simulink model "heli_day4_2"  (R2020b)
settings: Solver=ode1  StartTime=0.0  StopTime=20  FixedStep=0.002  RelTol=1e-3  EnableMultiTasking=on
PostLoadFcn:
  | qc_set_target_type(getConfigSet(bdroot, 'QUARC Default Target Configuration'));
undefined symbols (not defined in the file or in its folder): A_d, B_d, C_d, F, HIL, Joystick_gain_x, Joystick_gain_y, K, Q_d, qc_get_step_size, R_d
libraries: quarc_library x9
settings Model: SimulationMode=external  ExtModeTrigDuration=5000  Creator=Rchan  LastModifiedBy=endreeg
settings SolverCC: PositivePriorityOrder=on
settings DataIOCC: LimitDataPoints=on  SaveFormat=Array  SignalLoggingSaveFormat=ModelDataLogs  ReturnWorkspaceOutputs=off
settings OptimizationCC: ExpressionDepthLimit=2147483647  InitFltsAndDblsToZero=on  LifeSpan=inf
settings DebuggingCC: SaveWithParameterizedLinksMsg=none  UnderspecifiedInitializationDetection=Classic  MergeDetectMultiDrivingBlocksExec=none  SolverPrmCheckMsg=warning  MultiTaskDSMMsg=warning  MultiTaskCondExecSysMsg=none  FcnCallInpInsideContextMsg=warning  AllowSymbolicDim=off  StateNameClashWarn=warning  SFUnexpectedBacktrackingDiag=warning  SFNoUnconditionalDefaultTransitionDiag=warning  SFExecutionAtInitializationDiag=none  ArithmeticOperatorsInVariantConditions=warning
settings HardwareCC: ProdBitPerPointer=32  ProdBitPerSizeT=32  ProdBitPerPtrDiffT=32  ProdLargestAtomicFloat=None  ProdIntDivRoundTo=Undefined  ProdEndianess=Unspecified  ProdWordSize=32  ProdHWDeviceType=32-bit Generic
settings ModelReferenceCC: PropagateSignalLabelsOutOfModel=off
settings SFSimCC: SimUseLocalCustomCode=off  CustomCodeUndefinedFunction=UseInterfaceOnly
settings RTWCC: Description=QUARC Win64 Target  SystemTargetFile=quarc_win64.tlc  TemplateMakefile=quarc_default_tmf  RTWUseLocalCustomCode=off
settings CodeAppCC: StateflowObjectComments=on
settings GRTTargetCC: TargetLangStandard=C89/C90 (ANSI)  ParMdlRefBuildCompliant=off  CompOptLevelCompliant=off  CombineOutputUpdateFcns=off  MatFileLogging=off  GRTInterface=on  UseToolchainInfoCompliant=off  ExtMode=on  ExtModeMexFile=quarc_comm
settings ConfigComp: CovMetricSettings=dw  CovSaveCumulativeToWorkspaceVar=on  CovSaveSingleToWorkspaceVar=on  CovExternalEMLEnable=off  CovSFcnEnable=off

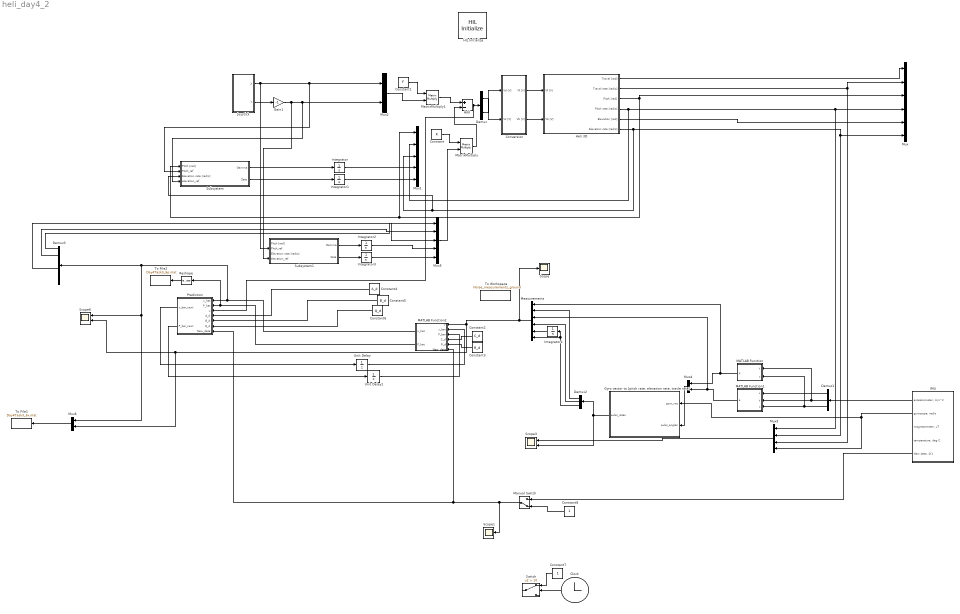
== system heli_day4_2 ==
  Add : Sum  Inputs=+-
  Clock : Clock
  Constant : Constant  Value=K
  Constant1 : Constant  Value=F
  Constant2 : Constant  Value=C_d
  Constant3 : Constant  Value=R_d
  Constant4 : Constant  Value=A_d
  Constant5 : Constant  Value=B_d
  Constant6 : Constant  Value=Q_d
  Constant7 : Constant
  Constant8 : Constant
  Conversion : Subsystem
  Demux : Demux  Outputs=2
  Demux1 : Demux  Outputs=3
  Demux2 : Demux  Outputs=3
  Demux3 : Demux  Outputs=6
  Gain1 : Gain  Gain=-1
  "Gyro vector to [pitch rate, elevation rate, travle rate]" : MATLAB Function  TreatAsAtomicUnit=on
  HIL Initialize : quarc_library/Data Acquisition/Generic/Configuration/HIL Initialize  Priority=-99  object_name=HIL-1  board_type=q8_usb  board_number=0  board_options=update_rate=normal;decimation=1  exclusive=off  active=off  hardware_clocks=[0:2]  clock_modes=[]  initial_clock_frequencies=[]  set_clock_params_at_start=off  set_clock_params_at_switch_in=off  set_clock_frequencies_at_start=off  set_clock_frequencies_at_switch_in=off  analog_input_channels=[0:7]  analog_input_configurations=[]  analog_input_maximums=10  analog_input_minimums=-10  set_analog_input_params_at_start=on  set_analog_input_params_at_switch_in=off  analog_output_channels=[0:7]  analog_output_maximums=10  analog_output_minimums=-10  initial_analog_outputs=[0]  final_analog_outputs=[0]  watchdog_analog_outputs=0  set_analog_output_params_at_start=on  set_analog_output_params_at_switch_in=off  set_analog_outputs_at_start=on  set_analog_outputs_at_switch_in=off  set_analog_outputs_at_terminate=on  set_analog_outputs_at_switch_out=off  set_analog_outputs_on_watchdog=off  digital_input_channels=[]  digital_output_channels=[]  digital_output_configuration=[]  initial_digital_outputs=[1]  final_digital_outputs=[1]  watchdog_digital_outputs=[1]  set_digital_output_params_at_start=off  set_digital_output_params_at_switch_in=off  set_digital_outputs_at_start=on  set_digital_outputs_at_switch_in=off  set_digital_outputs_at_terminate=on  set_digital_outputs_at_switch_out=off  set_digital_outputs_on_watchdog=off  encoder_channels=[0:7]  quadrature=[4]  encoder_filter_frequency=[]  initial_encoder_counts=[0]  set_encoder_params_at_start=on  set_encoder_params_at_switch_in=off  set_encoder_counts_at_start=on  set_encoder_counts_at_switch_in=off  pwm_channels=[0:7]  pwm_modes=0  pwm_frequency=99.532799999999995e6/4095  pwm_configuration=[0]  pwm_alignment=[0]  pwm_polarity=[1]  pwm_leading_deadband=[0]  pwm_trailing_deadband=[0]  initial_pwm_outputs=[0]  final_pwm_outputs=[0]  watchdog_pwm_outputs=[0]  set_pwm_params_at_start=on  set_pwm_params_at_switch_in=off  set_pwm_outputs_at_start=on  set_pwm_outputs_at_switch_in=off  set_pwm_outputs_at_terminate=on  set_pwm_outputs_at_switch_out=off  set_pwm_outputs_on_watchdog=off  other_output_channels=[]  initial_other_outputs=[]  final_other_outputs=[]  watchdog_other_outputs=[]  set_other_outputs_at_start=off  set_other_outputs_at_switch_in=off  set_other_outputs_at_terminate=off  set_other_outputs_at_switch_out=off  set_other_outputs_on_watchdog=off
  Heli 3D : Subsystem
  IMU : Subsystem
  Integrator{,1..4} (5 alike) : Integrator
  Joystick : Subsystem
  MATLAB Function : MATLAB Function  TreatAsAtomicUnit=on
  MATLAB Function1 : MATLAB Function  TreatAsAtomicUnit=on
  MATLAB Function2 : MATLAB Function  TreatAsAtomicUnit=on
  Manual Switch : ManualSwitch  CurrentSetting=0
  MatrixMultiply : Product  Multiplication=Matrix(*)
  MatrixMultiply1 : Product  Multiplication=Matrix(*)
  Measurements : Mux  Inputs=6
  Mux : Mux  Inputs=6
  Mux1 : Mux  Inputs=5
  Mux2 : Mux  Inputs=2
  Mux3 : Mux
  Mux4 : Mux  Inputs=2
  Mux5 : Mux  Inputs=5
  Mux6 : Mux  Inputs=2
  Prediction : MATLAB Function  TreatAsAtomicUnit=on
  Reshape : Reshape
  Scope : Scope
  Scope1 : Scope
  Scope3 : Scope  NumInputPorts=2
  Scope6 : Scope  NumInputPorts=2
  Subsystem : Subsystem
  Subsystem1 : Subsystem
  Switch : Switch  Criteria=u2 > Threshold  Threshold=10
  To File1 : ToFile  Filename=Day4Task3_6x.mat
  To File2 : ToFile  Filename=Day4Task3_6p.mat
  To Workspace : ToWorkspace  VariableName=Noise_measurements_ground  SampleTime=-1
  Unit Delay : UnitDelay  InitialCondition=[0,0,-0.5,0,0,0]  SampleTime=-1  HasFrameUpgradeWarning=on
  Unit Delay1 : UnitDelay  InitialCondition=eye(6)  SampleTime=-1  HasFrameUpgradeWarning=on
  wires:
  Heli 3D/1(Travel [rad]) -> Mux/1
  Heli 3D/2(Travel rate [rad/s]) -> Mux3/3, Mux/2
  Heli 3D/3(Pitch [rad]) -> Mux1/1, Subsystem/1(Pitch [rad]), Mux/3
  Heli 3D/4(Pitch rate [rad/s]) -> Mux3/1, Mux/4, Mux1/2
  Heli 3D/6(Elevation rate [rad/s]) -> Mux3/2, Mux/6, Mux1/3, Subsystem/3(Elevation rate [rad/s])
  Gain1/1 -> Mux2/2, Subsystem/4(elevation_ref), Subsystem1/4(elevation_ref)
  Joystick/2(Y) -> Gain1/1
  Demux/2 -> Conversion/1(Vd [V])
  MatrixMultiply/1 -> Add/2
  MatrixMultiply1/1 -> Add/1
  Constant/1 -> MatrixMultiply/1
  Constant1/1 -> MatrixMultiply1/1
  Mux2/1 -> MatrixMultiply1/2
  Demux/1 -> Conversion/2(Vs [V])
  Subsystem/1(Gamma) -> Integrator/1
  Integrator/1 -> Mux1/4
  Subsystem/2(Zeta) -> Integrator1/1
  Integrator1/1 -> Mux1/5
  Joystick/1(X) -> Mux2/1, Subsystem/2(Pitch_ref), Subsystem1/2(Pitch_ref)
  IMU/2("gyroscope, rad/s") -> "Gyro vector to [pitch rate, elevation rate, travle rate]"/1(gyro_vec), Mux3/4
  Mux3/1 -> Scope3/1
  IMU/1("accelerometer, m/s^2") -> Demux1/1
  Heli 3D/5(Elevation [rad]) -> Mux/5
  Mux4/1 -> "Gyro vector to [pitch rate, elevation rate, travle rate]"/2(euler_angles)
  MATLAB Function/1(p) -> Measurements/1, Mux4/1
  MATLAB Function1/1(e) -> Measurements/3, Mux4/2
  "Gyro vector to [pitch rate, elevation rate, travle rate]"/1(euler_rates) -> Demux2/1, Scope3/2
  Conversion/2(Vb [V]) -> Heli 3D/2(Vb [V])
  Conversion/1(Vf [V]) -> Heli 3D/1(Vf [V])
  Demux1/1 -> MATLAB Function1/1(x)
  Demux1/2 -> MATLAB Function/1(y), MATLAB Function1/2(y)
  Demux1/3 -> MATLAB Function/2(z), MATLAB Function1/3(z)
  Demux2/1 -> Measurements/2
  Demux2/2 -> Measurements/4
  Demux2/3 -> Measurements/6, Integrator4/1
  Subsystem1/1(Gamma) -> Integrator2/1
  Subsystem1/2(Zeta) -> Integrator3/1
  Integrator2/1 -> Mux5/4
  Integrator3/1 -> Mux5/5
  Demux3/1 -> Mux5/1
  Demux3/4 -> Mux5/3
  Demux3/2 -> Mux5/2
  Mux5/1 -> MatrixMultiply/2
  Mux6/1 -> To File1/1
  Integrator4/1 -> Measurements/5
  Measurements/1 -> Scope/1, MATLAB Function2/1(y), Mux6/2, Scope6/2
  Prediction/2(P_bar_next) -> Unit Delay1/1
  Constant2/1 -> MATLAB Function2/4(C_d)
  Constant3/1 -> MATLAB Function2/5(R_d)
  Unit Delay/1 -> MATLAB Function2/2(x_bar)
  Unit Delay1/1 -> MATLAB Function2/3(P_bar)
  Constant4/1 -> Prediction/4(A_d)
  Constant5/1 -> Prediction/5(B_d)
  Constant6/1 -> Prediction/6(Q_d)
  Prediction/1(x_bar_next) -> Unit Delay/1
  Add/1 -> Prediction/3(u), Demux/1
  MATLAB Function2/1(x_hat) -> Mux6/1, Scope6/1, Demux3/1, Prediction/1(x_hat)
  MATLAB Function2/2(P_hat) -> Reshape/1, Prediction/2(P_hat)
  Clock/1 -> Switch/2
  Constant7/1 -> Switch/1
  Constant8/1 -> Manual Switch/2
  IMU/5("New data, 0/1") -> Manual Switch/1
  Manual Switch/1 -> Scope1/1, Prediction/7(New_data), MATLAB Function2/6(New_data)
  Reshape/1 -> To File2/1

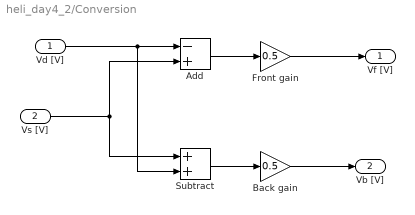
== system heli_day4_2/Conversion ==
  Vd [V] : Inport
  Vs [V] : Inport  Port=2
  Add : Sum  Inputs=-+
  Back gain : Gain  Gain=0.5
  Front gain : Gain  Gain=0.5
  Subtract : Sum
  Vf [V] : Outport
  Vb [V] : Outport  Port=2
  wires:
  Vd [V]/1 -> Subtract/2, Add/1
  Vs [V]/1 -> Add/2, Subtract/1
  Subtract/1 -> Back gain/1
  Back gain/1 -> Vb [V]/1
  Add/1 -> Front gain/1
  Front gain/1 -> Vf [V]/1

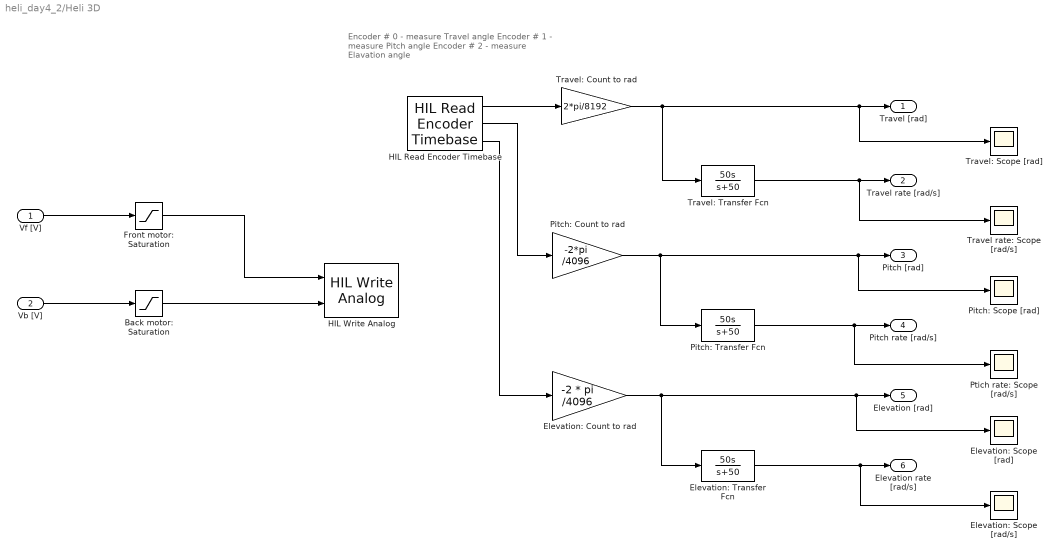
== system heli_day4_2/Heli 3D ==
  note: Encoder # 0 - measure Travel angle
      | Encoder # 1 - measure Pitch angle
      | Encoder # 2 - measure Elavation angle
  Vf [V] : Inport
  Vb [V] : Inport  Port=2
  Back motor: Saturation : Saturate  UpperLimit=5  LowerLimit=-5
  Elevation: Count to rad : Gain  Gain=-2 * pi /4096
  Elevation: Scope [rad/s] : Scope
  Elevation: Scope [rad] : Scope
  Elevation: Transfer Fcn : TransferFcn  Numerator=[50 0]  Denominator=[1 50]
  Front motor: Saturation : Saturate  UpperLimit=5  LowerLimit=-5
  HIL Read Encoder Timebase : quarc_library/Data Acquisition/Generic/Timebases/HIL Read Encoder Timebase  object_name=HIL-1  clock=0  channels=[0:2]  active=on  vector_output=off  data_type_mode=Inherit via back propagation  data_type=double  overflow_mode=Error on overflow  samples_in_buffer=max(ceil(1/qc_get_step_size), 1)
  HIL Write Analog : quarc_library/Data Acquisition/Generic/Immediate I//O/HIL Write Analog  object_name=HIL-1  channels=[0:1]  sample_time=-1  active=off  vector_input=off
  Pitch: Count to rad : Gain  Gain=-2*pi /4096
  Pitch: Scope [rad] : Scope
  Pitch: Transfer Fcn : TransferFcn  Numerator=[50 0]  Denominator=[1 50]
  Ptich rate: Scope [rad/s] : Scope
  Travel rate: Scope [rad/s] : Scope
  Travel: Count to rad : Gain  Gain=2*pi/8192
  Travel: Scope [rad] : Scope
  Travel: Transfer Fcn : TransferFcn  Numerator=[50 0]  Denominator=[1 50]
  Travel [rad] : Outport
  Travel rate [rad/s] : Outport  Port=2
  Pitch [rad] : Outport  Port=3
  Pitch rate [rad/s] : Outport  Port=4
  Elevation [rad] : Outport  Port=5
  Elevation rate [rad/s] : Outport  Port=6
  wires:
  HIL Read Encoder Timebase/1 -> Travel: Count to rad/1
  HIL Read Encoder Timebase/2 -> Pitch: Count to rad/1
  HIL Read Encoder Timebase/3 -> Elevation: Count to rad/1
  Travel: Count to rad/1 -> Travel: Scope [rad]/1, Travel [rad]/1, Travel: Transfer Fcn/1
  Travel: Transfer Fcn/1 -> Travel rate: Scope [rad/s]/1, Travel rate [rad/s]/1
  Pitch: Count to rad/1 -> Pitch: Transfer Fcn/1, Pitch: Scope [rad]/1, Pitch [rad]/1
  Pitch: Transfer Fcn/1 -> Ptich rate: Scope [rad/s]/1, Pitch rate [rad/s]/1
  Elevation: Count to rad/1 -> Elevation: Transfer Fcn/1, Elevation: Scope [rad]/1, Elevation [rad]/1
  Elevation: Transfer Fcn/1 -> Elevation: Scope [rad/s]/1, Elevation rate [rad/s]/1
  Vf [V]/1 -> Front motor: Saturation/1
  Vb [V]/1 -> Back motor: Saturation/1
  Front motor: Saturation/1 -> HIL Write Analog/1
  Back motor: Saturation/1 -> HIL Write Analog/2

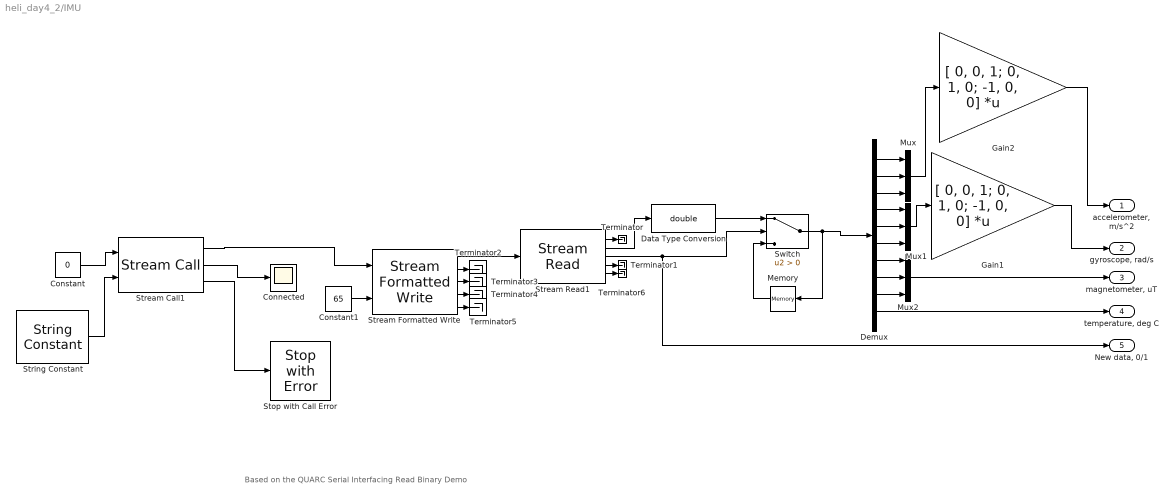
== system heli_day4_2/IMU ==
  note: Based on the QUARC Serial Interfacing Read Binary Demo
  Connected : Scope
  Constant : Constant  Value=0
  Constant1 : Constant  Value=65
  Data Type Conversion : DataTypeConversion  OutDataTypeStr=double
  Demux : Demux  Outputs=10
  Gain1 : Gain  Gain=[ 0, 0, 1; 0, 1, 0; -1, 0, 0]  Multiplication=Matrix(K*u) (u vector)
  Gain2 : Gain  Gain=[ 0, 0, 1; 0, 1, 0; -1, 0, 0]  Multiplication=Matrix(K*u) (u vector)
  Memory : Memory  InitialCondition=[0 0 0 0 0 0 0 0 0 0]
  Mux : Mux  Inputs=3
  Mux1 : Mux  Inputs=3
  Mux2 : Mux  Inputs=3
  Stop with Call Error : quarc_library/Sinks/Error Handling/Stop with Error  message_type=Interpret input as error code  message=Error occurred
      settings: SourceProductName=QUARC Targets
  Stream Call1 : quarc_library/Communications/Intermediate/Stream Call  uri_source=External input port  uri=serial://IMU:9?baud=115200,word=8,parity=none,stop=1,flow='none'  apply_uri_to_all_configs=on  send_buffer_size=8000  receive_buffer_size=8000  byte_order=little endian (Intel - LSB first)  sample_time=qc_get_step_size  non_blocking=on  active=off
      settings: SourceProductName=QUARC Targets
  Stream Formatted Write : quarc_library/Communications/Intermediate/Stream Formatted Write  format_string=%c\n  max_code_units=80  optimization=Minimizing latency
      settings: SourceProductName=QUARC Targets
  Stream Read1 : quarc_library/Communications/Intermediate/Stream Read  data_type=single  type_expr=BusObject  num_elements=10  receive_dims=off
      settings: SourceProductName=QUARC Targets
  String Constant : quarc_library/Strings/String Constant  string_value=qc_perform_substitutions('serial://IMU:%{PORT}?baud=115200,word=8,parity=none,stop=1')  evaluate_string=on  string_type=URI  max_length=255  sample_time=inf  variable_size=off
      settings: AttributesFormatString="\"serial://IMU:5?baud=115200,word=8,parity=none,stop=1\""  SourceProductName=QUARC Targets
  Switch : Switch  Criteria=u2 > Threshold
  Terminator{,1..6} (7 alike) : Terminator
  "accelerometer, m/s^2" : Outport
  "gyroscope, rad/s" : Outport  Port=2
  "magnetometer, uT" : Outport  Port=3
  "temperature, deg C" : Outport  Port=4
  "New data, 0/1" : Outport  Port=5
  wires:
  Switch/1 -> Memory/1, Demux/1
  Data Type Conversion/1 -> Switch/1
  Stream Read1/3 -> "New data, 0/1"/1, Switch/2
  Stream Formatted Write/1 -> Stream Read1/1
  Constant1/1 -> Stream Formatted Write/2
  Gain1/1 -> "gyroscope, rad/s"/1
  Gain2/1 -> "accelerometer, m/s^2"/1
  Stream Read1/4 -> Terminator1/1
  Demux/10 -> "temperature, deg C"/1
  Mux1/1 -> Gain1/1
  Stream Read1/2 -> Data Type Conversion/1
  Demux/7 -> Mux2/1
  Demux/8 -> Mux2/2
  Demux/9 -> Mux2/3
  Mux2/1 -> "magnetometer, uT"/1
  Demux/6 -> Mux1/3
  Demux/5 -> Mux1/2
  Demux/4 -> Mux1/1
  Mux/1 -> Gain2/1
  Demux/3 -> Mux/3
  Demux/1 -> Mux/1
  Demux/2 -> Mux/2
  Stream Read1/1 -> Terminator/1
  Stream Call1/1 -> Stream Formatted Write/1
  Constant/1 -> Stream Call1/1
  String Constant/1 -> Stream Call1/2
  Stream Call1/2 -> Connected/1
  Stream Call1/3 -> Stop with Call Error/1
  Memory/1 -> Switch/3
  Stream Formatted Write/2 -> Terminator2/1
  Stream Formatted Write/3 -> Terminator3/1
  Stream Formatted Write/4 -> Terminator4/1
  Stream Formatted Write/5 -> Terminator5/1
  Stream Read1/5 -> Terminator6/1

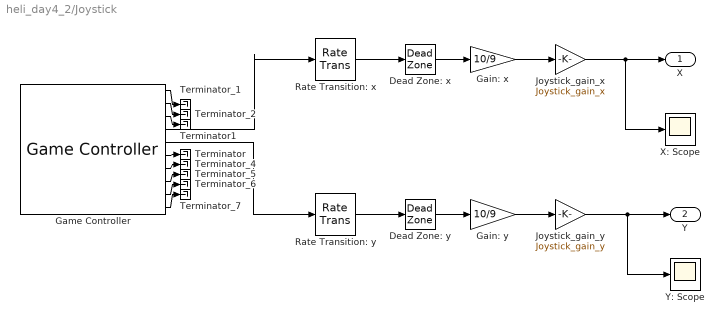
== system heli_day4_2/Joystick ==
  Dead Zone: x : DeadZone  LowerValue=-0.1  UpperValue=0.1  SaturateOnIntegerOverflow=on
  Dead Zone: y : DeadZone  LowerValue=-0.1  UpperValue=0.1  SaturateOnIntegerOverflow=on
  Gain: x : Gain  Gain=10/9
  Gain: y : Gain  Gain=10/9
  Game Controller : quarc_library/Devices/Peripherals/Target/Game Controller  controller=1  buffer_size=12  deadzone=[]  saturation=[]  sample_time=max(qc_get_step_size, 0.01)  auto_center=off  enabled=on
      settings: SourceProductName=QUARC Targets
  Joystick_gain_x : Gain  Gain=Joystick_gain_x
  Joystick_gain_y : Gain  Gain=Joystick_gain_y
  Rate Transition: x : RateTransition
  Rate Transition: y : RateTransition
  Terminator : Terminator
  Terminator1 : Terminator
  Terminator_{1..2,4..7} (6 alike) : Terminator
  X: Scope : Scope
  Y: Scope : Scope
  X : Outport
  Y : Outport  Port=2
  wires:
  Rate Transition: y/1 -> Dead Zone: y/1
  Rate Transition: x/1 -> Dead Zone: x/1
  Game Controller/5 -> Rate Transition: y/1
  Game Controller/4 -> Rate Transition: x/1
  Game Controller/1 -> Terminator_1/1
  Game Controller/2 -> Terminator_2/1
  Game Controller/7 -> Terminator_4/1
  Game Controller/8 -> Terminator_5/1
  Game Controller/9 -> Terminator_6/1
  Game Controller/10 -> Terminator_7/1
  Game Controller/3 -> Terminator1/1
  Game Controller/6 -> Terminator/1
  Dead Zone: x/1 -> Gain: x/1
  Dead Zone: y/1 -> Gain: y/1
  Gain: x/1 -> Joystick_gain_x/1
  Gain: y/1 -> Joystick_gain_y/1
  Joystick_gain_x/1 -> X/1, X: Scope/1
  Joystick_gain_y/1 -> Y: Scope/1, Y/1

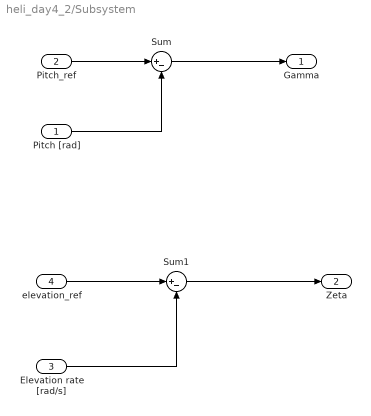
== system heli_day4_2/Subsystem ==
  Pitch [rad] : Inport
  Pitch_ref : Inport  Port=2
  Elevation rate [rad/s] : Inport  Port=3
  elevation_ref : Inport  Port=4
  Sum : Sum  Inputs=|+-
  Sum1 : Sum  Inputs=|+-
  Gamma : Outport
  Zeta : Outport  Port=2
  wires:
  Pitch_ref/1 -> Sum/1
  Sum/1 -> Gamma/1
  Pitch [rad]/1 -> Sum/2
  Sum1/1 -> Zeta/1
  elevation_ref/1 -> Sum1/1
  Elevation rate [rad/s]/1 -> Sum1/2

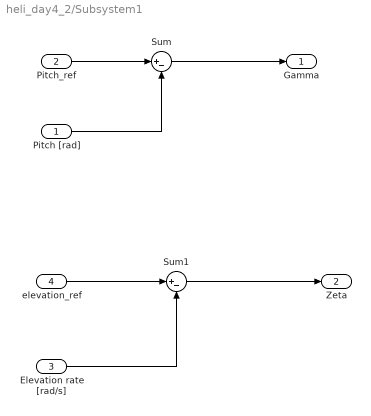
== system heli_day4_2/Subsystem1 ==
  Pitch [rad] : Inport
  Pitch_ref : Inport  Port=2
  Elevation rate [rad/s] : Inport  Port=3
  elevation_ref : Inport  Port=4
  Sum : Sum  Inputs=|+-
  Sum1 : Sum  Inputs=|+-
  Gamma : Outport
  Zeta : Outport  Port=2
  wires:
  Pitch_ref/1 -> Sum/1
  Sum/1 -> Gamma/1
  Pitch [rad]/1 -> Sum/2
  Sum1/1 -> Zeta/1
  elevation_ref/1 -> Sum1/1
  Elevation rate [rad/s]/1 -> Sum1/2

== matlab function heli_day4_2/Gyro vector to [pitch rate, elevation rate, travle rate] ==
  data: gyro_vec input; euler_rates output; euler_angles input
function euler_rates = gyro_vec_to_euler_rates(gyro_vec,euler_angles)
%#codegen
    phi = euler_angles(1);
    theta = euler_angles(2);


    T = [1, sin(phi)*tan(theta), cos(phi)*tan(theta);
         0, cos(phi),            -sin(phi);
         0, sin(phi)/cos(theta), cos(phi)/cos(theta)]; 
euler_rates = T*gyro_vec;

== matlab function heli_day4_2/MATLAB Function ==
  data: y input; p output; z input
function p = fcn(y, z)
if (z)
    p = atan(y/z);
else
    p=0;
end

== matlab function heli_day4_2/MATLAB Function1 ==
  data: x input; e output; y input; z input
function e = fcn(x, y, z)
if (z)
    e = atan(x/(sqrt(y^2+z^2)))+0.565;
else
    e=0;
end

== matlab function heli_day4_2/MATLAB Function2 ==
  data: y input; x_hat output; x_bar input; P_bar input; P_hat output; C_d input; R_d input; New_data input
function [x_hat,P_hat] = correction(y, x_bar, P_bar,C_d,R_d, New_data)
if New_data

    L_gain=P_bar*C_d'*inv(C_d*P_bar*C_d'+R_d);
    x_hat=x_bar+L_gain*(y-C_d*x_bar);
    P_hat=(eye(6)-L_gain*C_d)*P_bar*(eye(6)-L_gain*C_d)'+L_gain*R_d*L_gain';

else
    x_hat = x_bar;
    P_hat = P_bar;
end

end

== matlab function heli_day4_2/Prediction ==
  data: x_hat input; x_bar_next output; P_hat input; u input; A_d input; B_d input; Q_d input; P_bar_next output; New_data input
function [x_bar_next,P_bar_next] = prediction(x_hat, P_hat,u,A_d,B_d,Q_d, New_data)

if New_data
    x_bar_next=A_d*x_hat+B_d*u;
    P_bar_next=A_d*P_hat*A_d'+Q_d;
    
else
    x_bar_next = x_hat;
    P_bar_next = P_hat;
end
    
end
